simulink model "SimuLink1"  (R2023b)
settings: Solver=FixedStepAuto  StartTime=0.0  StopTime=10.0  FixedStep=0.5  MaxStep=0.5  RelTol=1e-9
settings Model: Creator=lyndo  LastModifiedBy=Cyrus Chavez

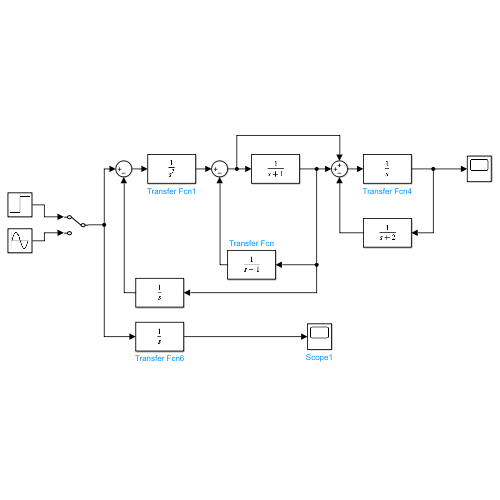
[thumbnail: Simulink's stored preview of the top-level diagram]
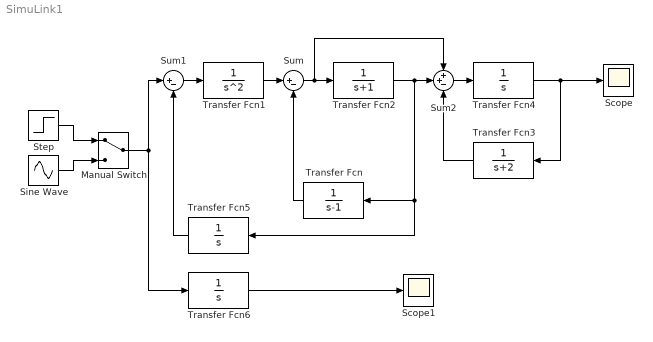
== system SimuLink1 ==
  Manual Switch : ManualSwitch
  Scope : Scope
  Scope1 : Scope
  Sine Wave : Sin  SampleTime=0
  Step : Step  SampleTime=0
  Sum : Sum  Inputs=|+-
  Sum1 : Sum  Inputs=|+-
  Sum2 : Sum  Inputs=++-
  Transfer Fcn : TransferFcn  Denominator=[1 -1]
  Transfer Fcn1 : TransferFcn  Denominator=[1 0 0]
  Transfer Fcn2 : TransferFcn  Denominator=[1 1]
  Transfer Fcn3 : TransferFcn  Denominator=[1 2]
  Transfer Fcn4 : TransferFcn  Denominator=[1 0]
  Transfer Fcn5 : TransferFcn  Denominator=[1 0]
  Transfer Fcn6 : TransferFcn  Denominator=[1 0]
  wires:
  Sum/1 -> Transfer Fcn2/1, Sum2/1
  Transfer Fcn2/1 -> Sum2/2, Transfer Fcn/1, Transfer Fcn5/1
  Transfer Fcn/1 -> Sum/2
  Transfer Fcn5/1 -> Sum1/2
  Sum2/1 -> Transfer Fcn4/1
  Transfer Fcn4/1 -> Transfer Fcn3/1, Scope/1
  Manual Switch/1 -> Sum1/1, Transfer Fcn6/1
  Step/1 -> Manual Switch/1
  Sine Wave/1 -> Manual Switch/2
  Sum1/1 -> Transfer Fcn1/1
  Transfer Fcn1/1 -> Sum/1
  Transfer Fcn3/1 -> Sum2/3
  Transfer Fcn6/1 -> Scope1/1
